simulink model "sampleModel47"  (R2021b)
settings: Solver=VariableStepAuto  StartTime=0.0  StopTime=10.0  RelTol=1e-3
undefined symbols (not defined in the file or in its folder): Newton, Raphson
libraries: simulink x6
settings Model: Creator=user  LastModifiedBy=user

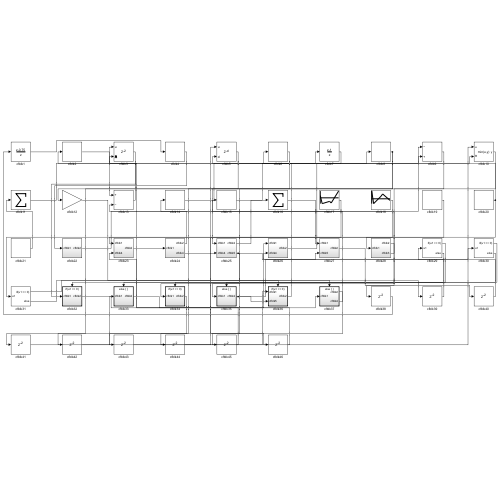
[thumbnail: Simulink's stored preview of the top-level diagram]
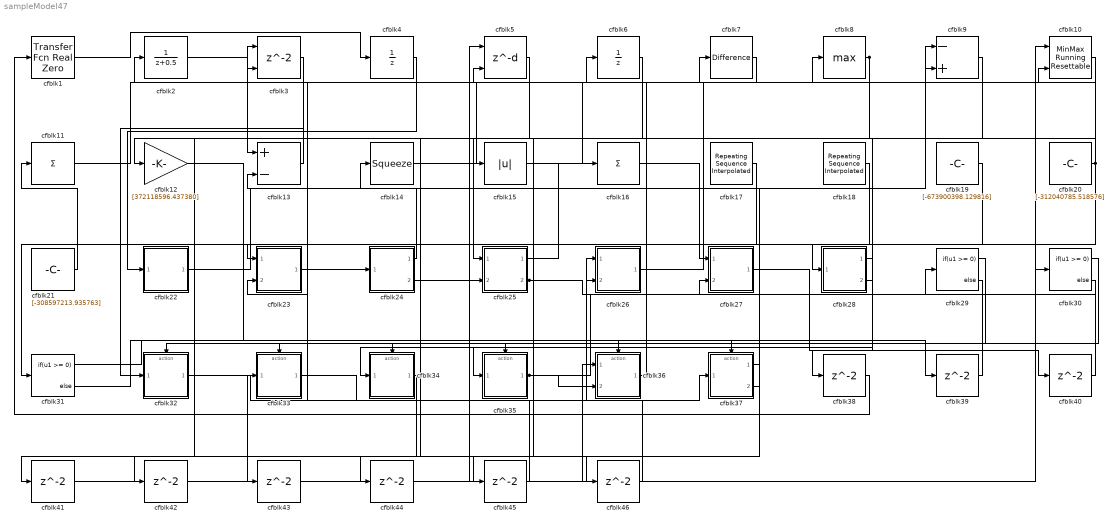
== system sampleModel47 ==
  cfblk1 : simulink/Discrete/Transfer Fcn Real Zero  ZeroZ=0.75  ICPrevInput=0.0  DoSatur=off
      settings: SourceProductBaseCode=SL
  cfblk10 : simulink/Math Operations/MinMax Running Resettable  Function=min  vinit=0.0
  cfblk11 : Sum  Inputs=+
  cfblk12 : Gain  Gain=[372118596.437380]
  cfblk13 : Sum  Inputs=+-
  cfblk14 : Squeeze
  cfblk15 : Abs
  cfblk16 : Sum  Inputs=+
  cfblk17 : simulink/Sources/Repeating Sequence Interpolated  OutValues=[279797014.763072, -684811340.754724, -420628156.321474, -602955982.973000, 863624828.386642]  TimeValues=[0 0.1 0.5 0.6 1].'  LookUpMeth=Use Input Below  tsamp=0.01  OutMin=[]  OutMax=[]  OutDataTypeStr=double  OutputDataTypeScalingMode=double  OutDataType=fixdt(0,8)  OutScaling=2^-10
  cfblk18 : simulink/Sources/Repeating Sequence Interpolated  OutValues=[905127054.246213, -565073033.898423, 290065765.026425, 572448864.892105, -199483780.497957]  TimeValues=[0 0.1 0.5 0.6 1].'  LookUpMeth=Use Input Above  tsamp=0.01  OutMin=[]  OutMax=[]  OutDataTypeStr=double  OutputDataTypeScalingMode=double  OutDataType=fixdt(0,8)  OutScaling=2^-10
  cfblk19 : Constant  Value=[-673900398.129816]  SampleTime=1
  cfblk2 : DiscreteTransferFcn  SampleTime=1
  cfblk20 : Constant  Value=[-312040785.518576]  SampleTime=1
  cfblk21 : Constant  Value=[-308597213.935763]  SampleTime=1
  cfblk22 : Subsystem
  cfblk23 : Subsystem
  cfblk24 : Subsystem
  cfblk25 : Subsystem
  cfblk26 : Subsystem
  cfblk27 : Subsystem
  cfblk28 : Subsystem
  cfblk29 : If  IfExpression=u1 >= 0  SampleTime=1
  cfblk3 : Delay  ShowEnablePort=on  SampleTime=1
      settings: InputPortMap=u0,e6
  cfblk30 : If  IfExpression=u1 >= 0  SampleTime=1
  cfblk31 : If  IfExpression=u1 >= 0  SampleTime=1
  cfblk32 : Subsystem  TreatAsAtomicUnit=on
  cfblk33 : Subsystem  TreatAsAtomicUnit=on
  cfblk34 : Subsystem  TreatAsAtomicUnit=on
  cfblk35 : Subsystem  TreatAsAtomicUnit=on
  cfblk36 : Subsystem  TreatAsAtomicUnit=on
  cfblk37 : Subsystem  TreatAsAtomicUnit=on
  cfblk{38..46} (9 alike) : Delay  SampleTime=1
  cfblk4 : UnitDelay  HasFrameUpgradeWarning=on
  cfblk5 : Delay  DelayLengthSource=Input port  SampleTime=1
      settings: InputPortMap=u0,p1
  cfblk6 : UnitDelay  HasFrameUpgradeWarning=on
  cfblk7 : simulink/Discrete/Difference  ICPrevInput=0.0  OutMin=[]  OutMax=[]  OutDataTypeStr=Inherit: Inherit via back propagation  OutDataType=fixdt(1, 16)  OutScaling=2^-10  DoSatur=off
  cfblk8 : MinMax  Function=max
  cfblk9 : Sum  Inputs=-+
  wires:
  cfblk8/1 -> cfblk12/1, cfblk35/1(cfblk1)
  cfblk25/1(cfblk2) -> cfblk16/1
  cfblk4/1 -> cfblk22/1(cfblk1)
  cfblk3/1 -> cfblk32/1(cfblk1)
  cfblk19/1 -> cfblk28/1(cfblk1)
  cfblk32/1(cfblk2) -> cfblk26/1(cfblk1)
  cfblk20/1 -> cfblk2/1, cfblk25/2(cfblk4)
  cfblk2/1 -> cfblk13/1
  cfblk35/1(cfblk2) -> cfblk10/1, cfblk36/2(cfblk5)
  cfblk13/1 -> cfblk3/1
  cfblk17/1 -> cfblk31/1
  cfblk24/1(cfblk2) -> cfblk3/2
  cfblk26/1(cfblk2) -> cfblk8/1
  cfblk16/1 -> cfblk27/1(cfblk1)
  cfblk22/1(cfblk2) -> cfblk9/1
  cfblk28/1(cfblk2) -> cfblk34/1(cfblk1)
  cfblk21/1 -> cfblk11/1
  cfblk33/1(cfblk2) -> cfblk37/1(cfblk1)
  cfblk10/1 -> cfblk25/1(cfblk1)
  cfblk7/1 -> cfblk5/2
  cfblk11/1 -> cfblk9/2
  cfblk28/2(cfblk3) -> cfblk14/1
  cfblk36/1(cfblk2) -> cfblk6/1
  cfblk18/1 -> cfblk23/1(cfblk1)
  cfblk1/1 -> cfblk4/1
  cfblk15/1 -> cfblk7/1
  cfblk14/1 -> cfblk10/2
  cfblk25/2(cfblk5) -> cfblk27/2(cfblk5), cfblk45/1
  cfblk37/2(cfblk4) -> cfblk15/1
  cfblk23/1(cfblk2) -> cfblk24/1(cfblk1)
  cfblk29/1 -> cfblk32/Action
  cfblk29/2 -> cfblk33/Action
  cfblk30/1 -> cfblk34/Action
  cfblk30/2 -> cfblk35/Action
  cfblk31/1 -> cfblk36/Action
  cfblk31/2 -> cfblk37/Action
  cfblk9/1 -> cfblk38/1
  cfblk38/1 -> cfblk1/1
  cfblk12/1 -> cfblk39/1
  cfblk39/1 -> cfblk26/2(cfblk4)
  cfblk27/1(cfblk2) -> cfblk40/1
  cfblk40/1 -> cfblk29/1
  cfblk37/1(cfblk2) -> cfblk41/1
  cfblk41/1 -> cfblk33/1(cfblk1)
  cfblk5/1 -> cfblk42/1
  cfblk42/1 -> cfblk36/1(cfblk1)
  cfblk34/1(cfblk2) -> cfblk43/1
  cfblk43/1 -> cfblk5/1
  cfblk6/1 -> cfblk44/1
  cfblk44/1 -> cfblk30/1
  cfblk45/1 -> cfblk13/2
  cfblk24/2(cfblk4) -> cfblk46/1
  cfblk46/1 -> cfblk23/2(cfblk4)

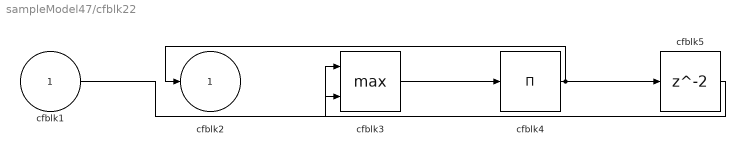
== system sampleModel47/cfblk22 ==
  cfblk1 : Inport
  cfblk3 : MinMax  Function=max  Inputs=2
  cfblk4 : Product  Inputs=*
  cfblk5 : Delay  SampleTime=1
  cfblk2 : Outport
  wires:
  cfblk4/1 -> cfblk2/1, cfblk5/1
  cfblk1/1 -> cfblk3/1
  cfblk3/1 -> cfblk4/1
  cfblk5/1 -> cfblk3/2

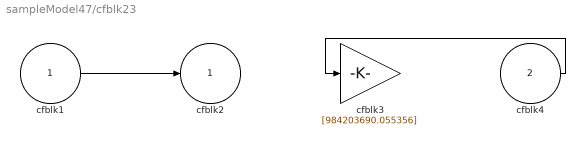
== system sampleModel47/cfblk23 ==
  cfblk1 : Inport
  cfblk4 : Inport  Port=2
  cfblk3 : Gain  Gain=[984203690.055356]
  cfblk2 : Outport
  wires:
  cfblk4/1 -> cfblk3/1
  cfblk1/1 -> cfblk2/1

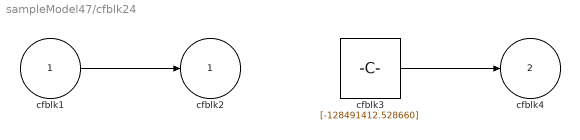
== system sampleModel47/cfblk24 ==
  cfblk1 : Inport
  cfblk3 : Constant  Value=[-128491412.528660]  SampleTime=1
  cfblk2 : Outport
  cfblk4 : Outport  Port=2
  wires:
  cfblk1/1 -> cfblk2/1
  cfblk3/1 -> cfblk4/1

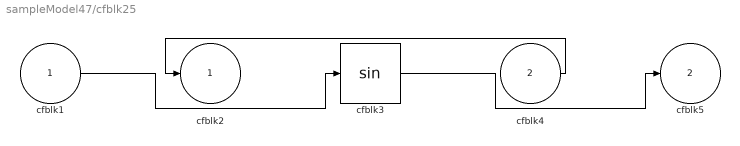
== system sampleModel47/cfblk25 ==
  cfblk1 : Inport
  cfblk4 : Inport  Port=2
  cfblk3 : Trigonometry
  cfblk2 : Outport
  cfblk5 : Outport  Port=2
  wires:
  cfblk4/1 -> cfblk2/1
  cfblk3/1 -> cfblk5/1
  cfblk1/1 -> cfblk3/1

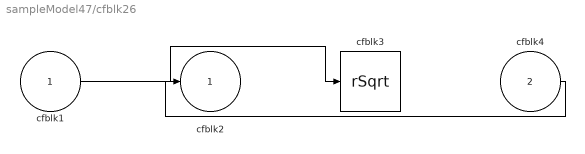
== system sampleModel47/cfblk26 ==
  cfblk1 : Inport
  cfblk4 : Inport  Port=2
  cfblk3 : Sqrt  Operator=rSqrt  AlgorithmType=Newton-Raphson  SaturateOnIntegerOverflow=on
  cfblk2 : Outport
  wires:
  cfblk1/1 -> cfblk3/1
  cfblk4/1 -> cfblk2/1

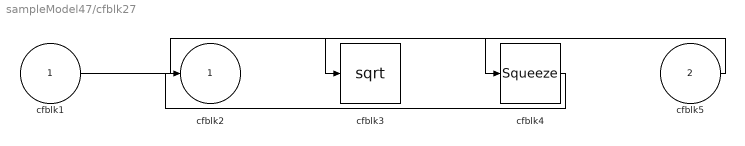
== system sampleModel47/cfblk27 ==
  cfblk1 : Inport
  cfblk5 : Inport  Port=2
  cfblk3 : Sqrt  SaturateOnIntegerOverflow=on
  cfblk4 : Squeeze
  cfblk2 : Outport
  wires:
  cfblk1/1 -> cfblk4/1
  cfblk4/1 -> cfblk2/1
  cfblk5/1 -> cfblk3/1

== system sampleModel47/cfblk28 ==
  cfblk1 : Inport
  cfblk2 : Outport
  cfblk3 : Outport  Port=2
  wires:
  cfblk1/1 -> cfblk2/1, cfblk3/1

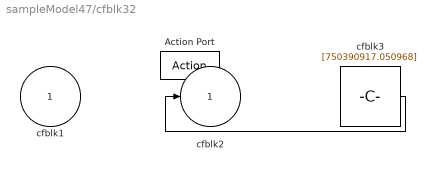
== system sampleModel47/cfblk32 ==
  cfblk1 : Inport
  Action Port : ActionPort  ActionPortLabel=if(u1 >= 0)
  cfblk3 : Constant  Value=[750390917.050968]  SampleTime=1
  cfblk2 : Outport
  wires:
  cfblk3/1 -> cfblk2/1

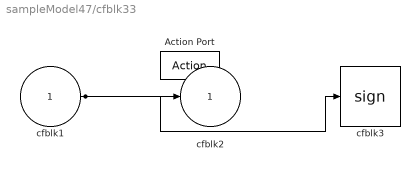
== system sampleModel47/cfblk33 ==
  cfblk1 : Inport
  Action Port : ActionPort  ActionPortLabel=else
  cfblk3 : Signum
  cfblk2 : Outport
  wires:
  cfblk1/1 -> cfblk2/1, cfblk3/1

== system sampleModel47/cfblk34 ==
  cfblk1 : Inport
  Action Port : ActionPort  ActionPortLabel=if(u1 >= 0)
  cfblk3 : Constant  Value=[60076696.691475]  SampleTime=1
  cfblk2 : Outport
  wires:
  cfblk1/1 -> cfblk2/1

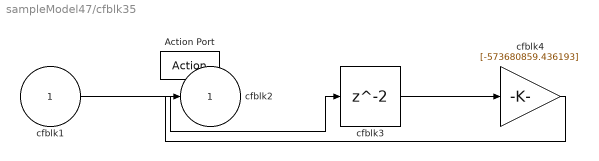
== system sampleModel47/cfblk35 ==
  cfblk1 : Inport
  Action Port : ActionPort  ActionPortLabel=else
  cfblk3 : Delay
  cfblk4 : Gain  Gain=[-573680859.436193]
  cfblk2 : Outport
  wires:
  cfblk3/1 -> cfblk4/1
  cfblk1/1 -> cfblk3/1
  cfblk4/1 -> cfblk2/1

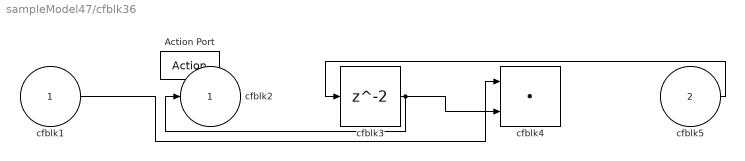
== system sampleModel47/cfblk36 ==
  cfblk1 : Inport
  cfblk5 : Inport  Port=2
  Action Port : ActionPort  ActionPortLabel=if(u1 >= 0)
  cfblk3 : Delay
  cfblk4 : DotProduct  InputSameDT=on  OutDataTypeStr=Inherit: Inherit via internal rule
  cfblk2 : Outport
  wires:
  cfblk3/1 -> cfblk2/1, cfblk4/2
  cfblk5/1 -> cfblk3/1
  cfblk1/1 -> cfblk4/1

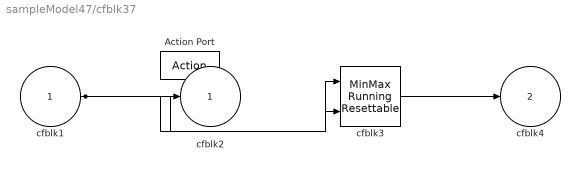
== system sampleModel47/cfblk37 ==
  cfblk1 : Inport
  Action Port : ActionPort  ActionPortLabel=else
  cfblk3 : simulink/Math Operations/MinMax Running Resettable  Function=min  vinit=0.0
  cfblk2 : Outport
  cfblk4 : Outport  Port=2
  wires:
  cfblk1/1 -> cfblk3/1, cfblk2/1, cfblk3/2
  cfblk3/1 -> cfblk4/1
